simulink model "mySimModel"  (R2024b)
settings: Solver=VariableStepAuto  StartTime=0.0  StopTime=10.0  RelTol=1e-3
settings Model: Creator=xinxing  LastModifiedBy=xinxing

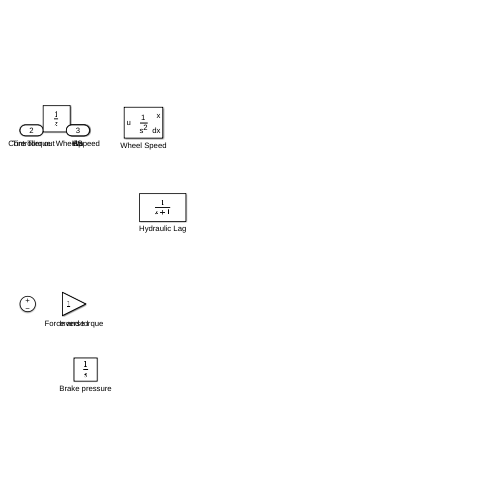
[thumbnail: Simulink's stored preview of the top-level diagram]
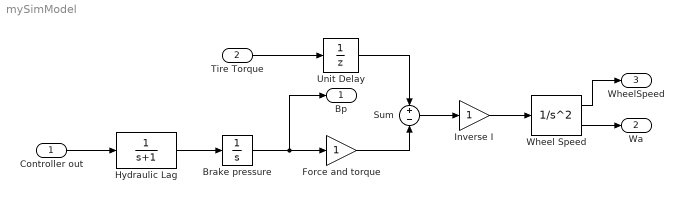
== system mySimModel ==
  Controller out : Inport
  Tire Torque : Inport  Port=2
  Brake pressure : Integrator
  Force and torque : Gain
  Hydraulic Lag : TransferFcn  Denominator=[1 1]
  Inverse I : Gain
  Sum : Sum  Inputs=+-
  Unit Delay : UnitDelay  SampleTime=-1  HasFrameUpgradeWarning=on
  Wheel Speed : SecondOrderIntegrator
  Bp : Outport
  Wa : Outport  Port=2
  WheelSpeed : Outport  Port=3
  wires:
  Wheel Speed/1 -> WheelSpeed/1
  Inverse I/1 -> Wheel Speed/1
  Sum/1 -> Inverse I/1
  Wheel Speed/2 -> Wa/1
  Brake pressure/1 -> Bp/1, Force and torque/1
  Force and torque/1 -> Sum/2
  Tire Torque/1 -> Unit Delay/1
  Unit Delay/1 -> Sum/1
  Hydraulic Lag/1 -> Brake pressure/1
  Controller out/1 -> Hydraulic Lag/1
